simulink model "vhs_fpga_rx_to_sdram_time_share_agc_cfo_4Chan"  (Simulink 7.1)
settings: Solver=FixedStepDiscrete  SolverMode=SingleTasking  StartTime=0.0  StopTime=120000  RelTol=1e-3
values from neighbouring files (symbols this model uses):
  Nfft = 64    [OFDM_Parameter.mat]
  Nguard = 16    [OFDM_Parameter.mat]
  Nofdm = 130    [OFDM_Parameter.mat]
  Nskip = 8    [OFDM_Parameter.mat]
undefined symbols (not defined in the file or in its folder): Fs, Sincos_Bits, Sincos_Len, Theta_Bits
libraries: xbsIndex_r4 x407, vhsadac_common_ob_fpgalib_v1_2_0 x18, misc_tools_fpgalib_v1_0_0 x6, rffe_fpgalib_v1_1_0 x1, rtdex_fpgalib_v1_1_0 x1
(part 3 of 5)

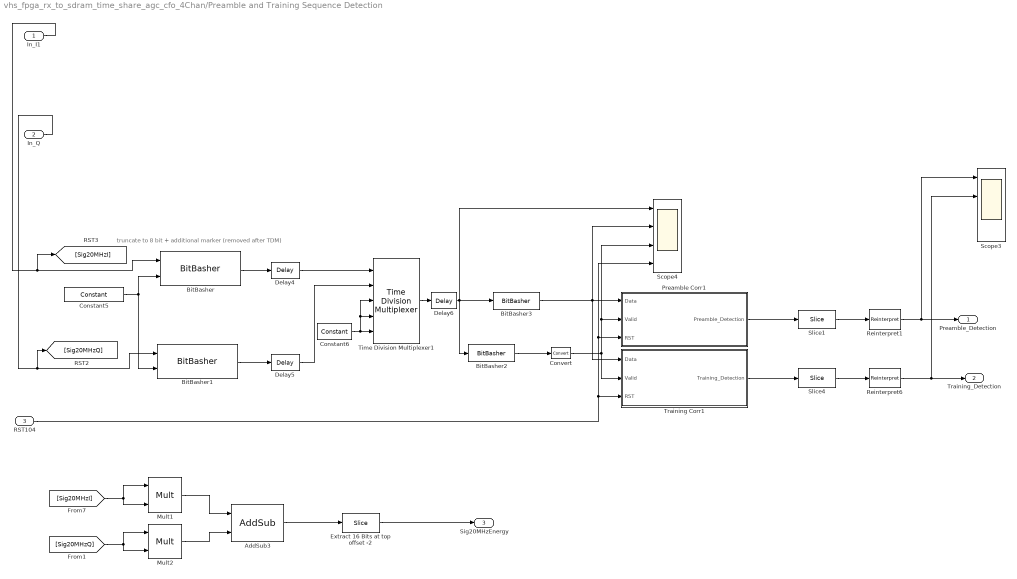
== system vhs_fpga_rx_to_sdram_time_share_agc_cfo_4Chan/Preamble and Training Sequence Detection ==
  note: truncate to 8 bit + additional marker (removed after TDM)
  In_I1 : Inport  OutDataType=sfix(16)  OutScaling=2^0
  In_Q : Inport  Port=2  OutDataType=sfix(16)  OutScaling=2^0
  RST104 : Inport  Port=3  OutDataType=sfix(16)  OutScaling=2^0
  "   Extract 16 Bits at top offset -2" : xbsIndex_r4/Slice  nbits=16  boolean_output=off  mode=Upper Bit Location + Width  bit1=-2  base1=MSB of Input  bit0=0  base0=LSB of Input  dbl_ovrd=off  block_type=slice
      settings: infoedit="Extracts a given range of bits from each input sample and presents it at the output.  The output type is ordinarily unsigned with binary point at zero, but can be Boolean when the slice is one bit wide.<P><P>Hardware notes: In hardware this block costs nothing."  block_version=10.1.3
  AddSub3 : xbsIndex_r4/AddSub  mode=Addition  use_carryin=off  use_carryout=off  en=off  latency=1  precision=Full  arith_type=Unsigned  n_bits=16  bin_pt=14  quantization=Truncate  overflow=Wrap  dbl_ovrd=off  use_behavioral_HDL=off  pipelined=off  use_rpm=on  hw_selection=Fabric  block_type=addsub
      settings: block_version=10.1.3
  BitBasher : xbsIndex_r4/BitBasher  bitexpr=|  display_expr=on  sr_1=1  arith_type1="Signed  (2's comp)"  bin_pt1=0  sr_2=2  arith_type2=Unsigned  bin_pt2=0  sr_3=3  arith_type3=Unsigned  bin_pt3=0  sr_4=4  arith_type4=Unsigned  bin_pt4=0  dbl_ovrd=off  block_type=bitbasher
      | <html><head><meta name="qrichtext" content="1" /><style type="text/css">
      | p, li { white-space: pre-wrap; }
      | </style></head><body style=" font-family:'MS Shell Dlg 2'; font-size:8.25pt; font-weight:400; font-style:normal;">
      | <p style=" margin-top:12px; margin-bottom:12px; margin-left:0px; margin-right:0px; -qt-block-indent:0; text-indent:0px; font-family:'MS Shell Dlg'; font-size:8pt;">a={b[13:6],c}</p></body></html>
      settings: block_version=10.1.3
  BitBasher1 : xbsIndex_r4/BitBasher  bitexpr=|  display_expr=on  sr_1=1  arith_type1="Signed  (2's comp)"  bin_pt1=0  sr_2=2  arith_type2=Unsigned  bin_pt2=0  sr_3=3  arith_type3=Unsigned  bin_pt3=0  sr_4=4  arith_type4=Unsigned  bin_pt4=0  dbl_ovrd=off  block_type=bitbasher
      | <html><head><meta name="qrichtext" content="1" /><style type="text/css">
      | p, li { white-space: pre-wrap; }
      | </style></head><body style=" font-family:'MS Shell Dlg 2'; font-size:8.25pt; font-weight:400; font-style:normal;">
      | <p style=" margin-top:12px; margin-bottom:12px; margin-left:0px; margin-right:0px; -qt-block-indent:0; text-indent:0px; font-family:'MS Shell Dlg'; font-size:8pt;">a={b[13:6],c}</p></body></html>
      settings: block_version=10.1.3
  BitBasher2 : xbsIndex_r4/BitBasher  bitexpr=|  display_expr=on  sr_1=1  arith_type1=Unsigned  bin_pt1=0  sr_2=2  arith_type2=Unsigned  bin_pt2=0  sr_3=3  arith_type3=Unsigned  bin_pt3=0  sr_4=4  arith_type4=Unsigned  bin_pt4=0  dbl_ovrd=off  block_type=bitbasher
      | <html><head><meta name="qrichtext" content="1" /><style type="text/css">
      | p, li { white-space: pre-wrap; }
      | </style></head><body style=" font-family:'MS Shell Dlg 2'; font-size:8.25pt; font-weight:400; font-style:normal;">
      | <p style=" margin-top:12px; margin-bottom:12px; margin-left:0px; margin-right:0px; -qt-block-indent:0; text-indent:0px; font-family:'MS Shell Dlg'; font-size:8pt;">a={b[0]}</p></body></html>
      settings: block_version=10.1.3
  BitBasher3 : xbsIndex_r4/BitBasher  bitexpr=|  display_expr=on  sr_1=1  arith_type1="Signed  (2's comp)"  bin_pt1=0  sr_2=2  arith_type2=Unsigned  bin_pt2=0  sr_3=3  arith_type3=Unsigned  bin_pt3=0  sr_4=4  arith_type4=Unsigned  bin_pt4=0  dbl_ovrd=off  block_type=bitbasher
      | <html><head><meta name="qrichtext" content="1" /><style type="text/css">
      | p, li { white-space: pre-wrap; }
      | </style></head><body style=" font-family:'MS Shell Dlg 2'; font-size:8.25pt; font-weight:400; font-style:normal;">
      | <p style=" margin-top:12px; margin-bottom:12px; margin-left:0px; margin-right:0px; -qt-block-indent:0; text-indent:0px; font-family:'MS Shell Dlg'; font-size:8pt;">a={b[8:1]}</p></body></html>
      settings: block_version=10.1.3
  Constant5 : xbsIndex_r4/Constant  arith_type=Unsigned  const=1  n_bits=1  bin_pt=0  explicit_period=on  period=5  equ=P=C  opselect=C  inp2=PCIN>>17  opr=+  inp1=P  carry=CIN  dbl_ovrd=off  block_type=constant
  Constant6 : xbsIndex_r4/Constant  arith_type=Signed (2's comp)  const=0  n_bits=9  bin_pt=0  explicit_period=on  period=5  equ=P=C  opselect=C  inp2=PCIN>>17  opr=+  inp1=P  carry=CIN  dbl_ovrd=off  block_type=constant
  Convert : xbsIndex_r4/Convert  arith_type=Boolean  n_bits=16  bin_pt=14  quantization=Truncate  overflow=Wrap  latency=0  dbl_ovrd=off  pipeline=off  block_type=convert
      settings: block_version=10.1.3
  Delay4 : xbsIndex_r4/Delay  en=off  latency=1  dbl_ovrd=off  reg_retiming=off  block_type=delay
  Delay5 : xbsIndex_r4/Delay  en=off  latency=1  dbl_ovrd=off  reg_retiming=off  block_type=delay
  Delay6 : xbsIndex_r4/Delay  en=off  latency=1  dbl_ovrd=off  reg_retiming=off  block_type=delay
  Mult1 : xbsIndex_r4/Mult  precision=Full  arith_type="Signed  (2's comp)"  n_bits=16  bin_pt=14  quantization=Truncate  overflow=Wrap  en=off  latency=3  dbl_ovrd=off  use_behavioral_HDL=off  use_embedded=on  opt=Speed  optimum_pipeline=off  pipeline=on  use_rpm=on  placement_style=Triangular  block_type=mult
      settings: infoedit=Hardware notes: To use the internal pipeline stage of the dedicated multiplier you must select 'Pipeline for maximum performance'.  block_version=10.1.3
  Mult2 : xbsIndex_r4/Mult  precision=Full  arith_type="Signed  (2's comp)"  n_bits=16  bin_pt=14  quantization=Truncate  overflow=Wrap  en=off  latency=3  dbl_ovrd=off  use_behavioral_HDL=off  use_embedded=on  opt=Speed  optimum_pipeline=off  pipeline=on  use_rpm=on  placement_style=Triangular  block_type=mult
      settings: infoedit=Hardware notes: To use the internal pipeline stage of the dedicated multiplier you must select 'Pipeline for maximum performance'.  block_version=10.1.3
  Preamble Corr1 : Subsystem
  Reinterpret1 : xbsIndex_r4/Reinterpret  force_arith_type=on  arith_type=Unsigned  force_bin_pt=on  bin_pt=0  block_type=reinterpret
      settings: infoedit="Changes signal type without altering the binary representation.   You can changed the signal between signed and unsigned, and relocate the binary point.<P><P>Hardware notes: In hardware this block costs nothing.<P><P>Example:  Suppose the input is 6 bits wide, signed, with 2 fractional bits, and the output is forced to unsigned with 0 fractional bits.  Then an input of -2.0 (1110.00 in binary 2's complement) becomes an output of 56 (111000 in binary)."  block_version=10.1.3
  Reinterpret6 : xbsIndex_r4/Reinterpret  force_arith_type=on  arith_type=Unsigned  force_bin_pt=on  bin_pt=0  block_type=reinterpret
      settings: infoedit="Changes signal type without altering the binary representation.   You can changed the signal between signed and unsigned, and relocate the binary point.<P><P>Hardware notes: In hardware this block costs nothing.<P><P>Example:  Suppose the input is 6 bits wide, signed, with 2 fractional bits, and the output is forced to unsigned with 0 fractional bits.  Then an input of -2.0 (1110.00 in binary 2's complement) becomes an output of 56 (111000 in binary)."  block_version=10.1.3
  Scope3 : Scope  NumInputPorts=4
      settings: YMin=-5~-5~-5~-5  YMax=5~5~5~5  SaveName=ScopeData5  MaxDataPoints=500000  SampleInput=on
  Scope4 : Scope  NumInputPorts=4
      settings: YMin=-300~-150~0~-1  YMax=200~100~1~1  SaveName=ScopeData10  MaxDataPoints=500000
  Slice1 : xbsIndex_r4/Slice  nbits=16  boolean_output=off  mode=Upper Bit Location + Width  bit1=-8  base1=MSB of Input  bit0=0  base0=LSB of Input  dbl_ovrd=off  block_type=slice
      settings: infoedit="Extracts a given range of bits from each input sample and presents it at the output.  The output type is ordinarily unsigned with binary point at zero, but can be Boolean when the slice is one bit wide.<P><P>Hardware notes: In hardware this block costs nothing."  block_version=10.1.3
  Slice4 : xbsIndex_r4/Slice  nbits=16  boolean_output=off  mode=Upper Bit Location + Width  bit1=-7  base1=MSB of Input  bit0=0  base0=LSB of Input  dbl_ovrd=off  block_type=slice
      settings: infoedit="Extracts a given range of bits from each input sample and presents it at the output.  The output type is ordinarily unsigned with binary point at zero, but can be Boolean when the slice is one bit wide.<P><P>Hardware notes: In hardware this block costs nothing."  block_version=10.1.3
  Time Division Multiplexer1 : xbsIndex_r4/Time Division Multiplexer  inputs=5  vin=off  dbl_ovrd=off  explicit_period=off  period=1  block_type=tdm
      settings: infoedit="Multiple inputs are sampled and  presented serially at the output."  block_version=10.1.3
  Training Corr1 : Subsystem
  Preamble_Detection : Outport  OutDataType=sfix(16)  OutScaling=2^0
  Training_Detection : Outport  Port=2  OutDataType=sfix(16)  OutScaling=2^0
  Sig20MHzEnergy : Outport  Port=3  OutDataType=sfix(16)  OutScaling=2^0
  wires:
  In_Q/1 -> BitBasher1/1, [Sig20MHzQ]
  In_I1/1 -> BitBasher/1, [Sig20MHzI]
  [Sig20MHzI] -> Mult1/1, Mult1/2
  [Sig20MHzQ] -> Mult2/2, Mult2/1
  Mult1/1 -> AddSub3/1
  Mult2/1 -> AddSub3/2
  AddSub3/1 -> "   Extract 16 Bits at top offset -2"/1
  "   Extract 16 Bits at top offset -2"/1 -> Sig20MHzEnergy/1
  Time Division Multiplexer1/1 -> Delay6/1
  Constant6/1 -> Time Division Multiplexer1/5, Time Division Multiplexer1/4, Time Division Multiplexer1/3
  BitBasher2/1 -> Convert/1
  Constant5/1 -> BitBasher/2, BitBasher1/2
  BitBasher1/1 -> Delay5/1
  BitBasher3/1 -> Preamble Corr1/1(Data), Training Corr1/1(Data), Scope4/2
  BitBasher/1 -> Delay4/1
  Convert/1 -> Training Corr1/2(Valid), Preamble Corr1/2(Valid), Scope4/3
  Preamble Corr1/1(Preamble_Detection) -> Slice1/1
  Slice1/1 -> Reinterpret1/1
  Delay4/1 -> Time Division Multiplexer1/1
  Delay5/1 -> Time Division Multiplexer1/2
  Delay6/1 -> BitBasher3/1, BitBasher2/1, Scope4/1
  Slice4/1 -> Reinterpret6/1
  Training Corr1/1(Training_Detection) -> Slice4/1
  Reinterpret6/1 -> Training_Detection/1, Scope3/2
  Reinterpret1/1 -> Preamble_Detection/1, Scope3/1
  RST104/1 -> Training Corr1/3(RST), Preamble Corr1/3(RST), Scope4/4

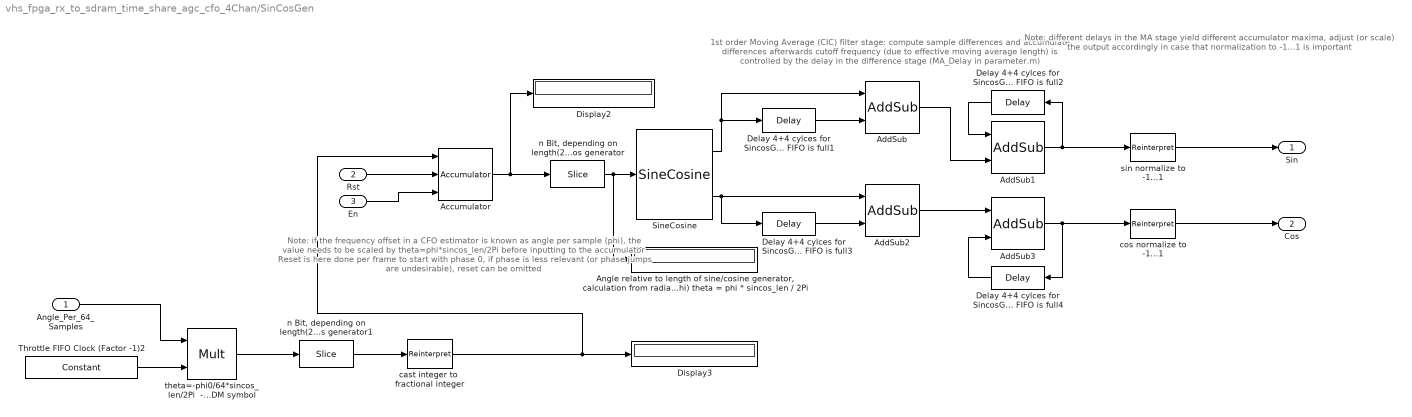
== system vhs_fpga_rx_to_sdram_time_share_agc_cfo_4Chan/SinCosGen ==
  note: 1st order Moving Average (CIC) filter stage:
      | compute sample differences and accumulate differences afterwards
      | cutoff frequency (due to effective moving average length) is
      | controlled by the delay in the difference stage (MA_Delay in parameter.m)
  note: Note: if the frequency offset in a CFO estimator
      | is known as angle per sample (phi),
      | the value needs to be scaled by
      | theta=phi*sincos_len/2Pi
      | before inputting to the accumulator
      | Reset is here done per frame to start with phase 0,
      | if phase is less relevant (or phase jumps are undesirable),
      | reset can be omitted
  note: Note: different delays in the MA stage yield different
      | accumulator maxima, adjust (or scale) the output accordingly
      | in case that normalization to -1...1 is important
  Angle_Per_64_Samples : Inport
  Rst : Inport  Port=2
  En : Inport  Port=3
  Accumulator : xbsIndex_r4/Accumulator  operation=Add  n_bits=Theta_Bits+Sincos_Bits+1  overflow=Wrap  scale=1  rst=on  hasbypass=off  en=on  dbl_ovrd=off  use_behavioral_HDL=on  implementation=Fabric  block_type=accum
      settings: infoedit="Adder or subtractor-based accumulator.   Output type and binary point position match the input.<P><P>Hardware notes: When \"Reinitialize with input 'b' on reset\" is selected, the accumulator is forced to run at the system rate even if the input 'b' is running at a slower rate."  block_version=10.1.3
  AddSub : xbsIndex_r4/AddSub  mode=Subtraction  use_carryin=off  use_carryout=off  en=off  latency=0  precision=Full  arith_type=Unsigned  n_bits=16  bin_pt=14  quantization=Truncate  overflow=Wrap  dbl_ovrd=off  use_behavioral_HDL=off  pipelined=off  use_rpm=on  hw_selection=Fabric  block_type=addsub
      settings: block_version=10.1.3
  AddSub1 : xbsIndex_r4/AddSub  mode=Addition  use_carryin=off  use_carryout=off  en=off  latency=0  precision=User Defined  arith_type="Signed  (2's comp)"  n_bits=16  bin_pt=8  quantization=Truncate  overflow=Wrap  dbl_ovrd=off  use_behavioral_HDL=off  pipelined=off  use_rpm=on  hw_selection=Fabric  block_type=addsub
      settings: block_version=10.1.3
  AddSub2 : xbsIndex_r4/AddSub  mode=Subtraction  use_carryin=off  use_carryout=off  en=off  latency=0  precision=Full  arith_type=Unsigned  n_bits=16  bin_pt=14  quantization=Truncate  overflow=Wrap  dbl_ovrd=off  use_behavioral_HDL=off  pipelined=off  use_rpm=on  hw_selection=Fabric  block_type=addsub
      settings: block_version=10.1.3
  AddSub3 : xbsIndex_r4/AddSub  mode=Addition  use_carryin=off  use_carryout=off  en=off  latency=0  precision=User Defined  arith_type="Signed  (2's comp)"  n_bits=16  bin_pt=8  quantization=Truncate  overflow=Wrap  dbl_ovrd=off  use_behavioral_HDL=off  pipelined=off  use_rpm=on  hw_selection=Fabric  block_type=addsub
      settings: block_version=10.1.3
  "Angle relative to length of sine/cosine generator, calculation from radians (phi) theta = phi * sincos_len / 2Pi" : Display
  Delay 4+4 cylces for SincosGen (Counter+Mult+SinCos latencies)  but stop immediately when FIFO is full1 : xbsIndex_r4/Delay  en=off  latency=MA_Delay  dbl_ovrd=off  reg_retiming=off  block_type=delay
  Delay 4+4 cylces for SincosGen (Counter+Mult+SinCos latencies)  but stop immediately when FIFO is full2 : xbsIndex_r4/Delay  Orientation=left  en=off  latency=1  dbl_ovrd=off  reg_retiming=off  block_type=delay
  Delay 4+4 cylces for SincosGen (Counter+Mult+SinCos latencies)  but stop immediately when FIFO is full3 : xbsIndex_r4/Delay  en=off  latency=MA_Delay  dbl_ovrd=off  reg_retiming=off  block_type=delay
  Delay 4+4 cylces for SincosGen (Counter+Mult+SinCos latencies)  but stop immediately when FIFO is full4 : xbsIndex_r4/Delay  Orientation=left  en=off  latency=1  dbl_ovrd=off  reg_retiming=off  block_type=delay
  Display2 : Display
  Display3 : Display
  SineCosine : xbsIndex_r4/SineCosine  mode=Sine and Cosine  neg_sin=off  neg_cos=off  n_bits=10  sym_output=on  en=off  latency=Sincos_Latency  dbl_ovrd=off  explicit_period=on  period=FreqDivider  mem_type=Distributed Memory  pipeline=off  use_rpm=on  block_type=sincos
      settings: block_version=10.1.3
  Throttle FIFO Clock (Factor -1)2 : xbsIndex_r4/Constant  arith_type=Signed (2's comp)  const=-1/64*Sincos_Len/(2*pi)  n_bits=32  bin_pt=28  explicit_period=on  period=5  equ=P=C  opselect=C  inp2=PCIN>>17  opr=+  inp1=P  carry=CIN  dbl_ovrd=off  block_type=constant
  cast integer to  fractional integer : xbsIndex_r4/Reinterpret  force_arith_type=on  arith_type="Signed  (2's comp)"  force_bin_pt=on  bin_pt=Theta_Bits  block_type=reinterpret
      settings: infoedit="Changes signal type without altering the binary representation.   You can changed the signal between signed and unsigned, and relocate the binary point.<P><P>Hardware notes: In hardware this block costs nothing.<P><P>Example:  Suppose the input is 6 bits wide, signed, with 2 fractional bits, and the output is forced to unsigned with 0 fractional bits.  Then an input of -2.0 (1110.00 in binary 2's complement) becomes an output of 56 (111000 in binary)."  block_version=10.1.3
  cos normalize to -1...1 : xbsIndex_r4/Reinterpret  force_arith_type=on  arith_type="Signed  (2's comp)"  force_bin_pt=on  bin_pt=14  block_type=reinterpret
      settings: infoedit="Changes signal type without altering the binary representation.   You can changed the signal between signed and unsigned, and relocate the binary point.<P><P>Hardware notes: In hardware this block costs nothing.<P><P>Example:  Suppose the input is 6 bits wide, signed, with 2 fractional bits, and the output is forced to unsigned with 0 fractional bits.  Then an input of -2.0 (1110.00 in binary 2's complement) becomes an output of 56 (111000 in binary)."  block_version=10.1.3
  "n Bit, depending on length(2^n) of sincos generator" : xbsIndex_r4/Slice  nbits=Sincos_Bits  boolean_output=off  mode=Lower Bit Location + Width  bit1=0  base1=MSB of Input  bit0=Theta_Bits  base0=LSB of Input  dbl_ovrd=off  block_type=slice
      settings: infoedit="Extracts a given range of bits from each input sample and presents it at the output.  The output type is ordinarily unsigned with binary point at zero, but can be Boolean when the slice is one bit wide.<P><P>Hardware notes: In hardware this block costs nothing."  block_version=10.1.3
  "n Bit, depending on length(2^n) of sincos generator1" : xbsIndex_r4/Slice  nbits=32  boolean_output=off  mode=Upper Bit Location + Width  bit1=0  base1=MSB of Input  bit0=Theta_Bits  base0=LSB of Input  dbl_ovrd=off  block_type=slice
      settings: infoedit="Extracts a given range of bits from each input sample and presents it at the output.  The output type is ordinarily unsigned with binary point at zero, but can be Boolean when the slice is one bit wide.<P><P>Hardware notes: In hardware this block costs nothing."  block_version=10.1.3
  sin normalize to -1...1 : xbsIndex_r4/Reinterpret  force_arith_type=on  arith_type="Signed  (2's comp)"  force_bin_pt=on  bin_pt=14  block_type=reinterpret
      settings: infoedit="Changes signal type without altering the binary representation.   You can changed the signal between signed and unsigned, and relocate the binary point.<P><P>Hardware notes: In hardware this block costs nothing.<P><P>Example:  Suppose the input is 6 bits wide, signed, with 2 fractional bits, and the output is forced to unsigned with 0 fractional bits.  Then an input of -2.0 (1110.00 in binary 2's complement) becomes an output of 56 (111000 in binary)."  block_version=10.1.3
  "theta=-phi0/64*sincos_len/2Pi  -> /64: CFO is for a distance of 64 samples between guard interval and main OFDM symbol" : xbsIndex_r4/Mult  precision=Full  arith_type="Signed  (2's comp)"  n_bits=16  bin_pt=14  quantization=Truncate  overflow=Wrap  en=off  latency=3  dbl_ovrd=off  use_behavioral_HDL=off  use_embedded=on  opt=Speed  optimum_pipeline=off  pipeline=on  use_rpm=on  placement_style=Triangular  block_type=mult
      settings: infoedit=Hardware notes: To use the internal pipeline stage of the dedicated multiplier you must select 'Pipeline for maximum performance'.  block_version=10.1.3
  Sin : Outport
  Cos : Outport  Port=2
  wires:
  "n Bit, depending on length(2^n) of sincos generator"/1 -> SineCosine/1, "Angle relative to length of sine/cosine generator, calculation from radians (phi) theta = phi * sincos_len / 2Pi"/1
  SineCosine/1 -> Delay 4+4 cylces for SincosGen (Counter+Mult+SinCos latencies)  but stop immediately when FIFO is full1/1, AddSub/1
  SineCosine/2 -> AddSub2/1, Delay 4+4 cylces for SincosGen (Counter+Mult+SinCos latencies)  but stop immediately when FIFO is full3/1
  Accumulator/1 -> "n Bit, depending on length(2^n) of sincos generator"/1, Display2/1
  cast integer to  fractional integer/1 -> Display3/1, Accumulator/1
  AddSub1/1 -> Delay 4+4 cylces for SincosGen (Counter+Mult+SinCos latencies)  but stop immediately when FIFO is full2/1, sin normalize to -1...1/1
  Delay 4+4 cylces for SincosGen (Counter+Mult+SinCos latencies)  but stop immediately when FIFO is full2/1 -> AddSub1/1
  Delay 4+4 cylces for SincosGen (Counter+Mult+SinCos latencies)  but stop immediately when FIFO is full3/1 -> AddSub2/2
  AddSub2/1 -> AddSub3/1
  AddSub3/1 -> Delay 4+4 cylces for SincosGen (Counter+Mult+SinCos latencies)  but stop immediately when FIFO is full4/1, cos normalize to -1...1/1
  Delay 4+4 cylces for SincosGen (Counter+Mult+SinCos latencies)  but stop immediately when FIFO is full4/1 -> AddSub3/2
  AddSub/1 -> AddSub1/2
  Delay 4+4 cylces for SincosGen (Counter+Mult+SinCos latencies)  but stop immediately when FIFO is full1/1 -> AddSub/2
  Rst/1 -> Accumulator/2
  Throttle FIFO Clock (Factor -1)2/1 -> "theta=-phi0/64*sincos_len/2Pi  -> /64: CFO is for a distance of 64 samples between guard interval and main OFDM symbol"/2
  "theta=-phi0/64*sincos_len/2Pi  -> /64: CFO is for a distance of 64 samples between guard interval and main OFDM symbol"/1 -> "n Bit, depending on length(2^n) of sincos generator1"/1
  "n Bit, depending on length(2^n) of sincos generator1"/1 -> cast integer to  fractional integer/1
  Angle_Per_64_Samples/1 -> "theta=-phi0/64*sincos_len/2Pi  -> /64: CFO is for a distance of 64 samples between guard interval and main OFDM symbol"/1
  sin normalize to -1...1/1 -> Sin/1
  cos normalize to -1...1/1 -> Cos/1
  En/1 -> Accumulator/3

== system vhs_fpga_rx_to_sdram_time_share_agc_cfo_4Chan/two times  long preamble detection ==
  note: original delay: (Nfft+Nguard)
      | due to shortened Training Correlator: Nfft-16
  Preamble Detection : Inport  OutDataType=sfix(16)  OutScaling=2^0
  Training Detection : Inport  Port=2  OutDataType=sfix(16)  OutScaling=2^0
  Delay1 : xbsIndex_r4/Delay  en=off  latency=48  dbl_ovrd=off  reg_retiming=off  block_type=delay
      settings: block_version=9.2.00
  Edge detector : misc_tools_fpgalib_v1_0_0/Edge detector  Tag=LYR_FPGA_MISC_EDGE_DETECTOR  Description=Lyrtech block  SystemSampleTime=-1  edge_detect=Rising  and_latency=0
  Expression6 : xbsIndex_r4/Expression  expression=a & b  align_bp=on  en=off  latency=0  precision=Full  arith_type=Unsigned  n_bits=16  bin_pt=0  dbl_ovrd=off  block_type=expr
      settings: block_version=10.1.3
  Detected : Outport  OutDataType=sfix(16)  OutScaling=2^0
  wires:
  Preamble Detection/1 -> Delay1/1
  Expression6/1 -> Edge detector/1
  Edge detector/1 -> Detected/1
  Training Detection/1 -> Expression6/2
  Delay1/1 -> Expression6/1

== system vhs_fpga_rx_to_sdram_time_share_agc_cfo_4Chan/CFO Estimate - triggered by WRITE_STATE going high/CORDIC ATAN1 ==
  note: The CORDIC algorithm is implemented in 3 steps.
      |
      | Step 1: Coarse Angle Rotation.  The algorithm converges only for angles between -pi/2 and pi/2, so if x < zero, the input vector is reflected
      | to the 1st or 3rd quadrant by making the x-coordinate non-negative.
      |
      | Step 2: Fine Angle Rotation.  For rectangular-to-polar conversion, the resulting vector is rotated through progressively smaller angles, such that y goes
      | to zero. In the i-th stage, the angular rotation is by either +/- atan(1/2^i), depending on whether or not its input y is less than or greater than zero.
      |
      | Step 3: Angle Correction. If there was a reflection applied in Step 1, this step applies the appropriate angle correction by subtracting it from +/- pi.
  x : Inport  OutDataType=sfix(16)  OutScaling=2^0
  y : Inport  Port=2  OutDataType=sfix(16)  OutScaling=2^0
  CORDIC  Pipe Balance : xbsIndex_r4/Delay  en=off  latency=sum(pipeline)  dbl_ovrd=off  reg_retiming=off  block_type=delay
      settings: infoedit="Delay line having  configurable length.<P><P>Hardware notes: A delay line is a chain, each link of which is an SRL16 followed by a flip-flop. If register retiming is enabled, the delay line is a chain of flip-flops."  xl_area=[0, 0, 0, 0, 0, 0, 0]  block_version=VER_STRING_GOES_HERE
  CORDIC  Pipe Balance1 : xbsIndex_r4/Delay  en=off  latency=sum(pipeline)+1  dbl_ovrd=off  reg_retiming=off  block_type=delay
      settings: infoedit="Delay line having  configurable length.<P><P>Hardware notes: A delay line is a chain, each link of which is an SRL16 followed by a flip-flop. If register retiming is enabled, the delay line is a chain of flip-flops."  xl_area=[0, 0, 0, 0, 0, 0, 0]  block_version=VER_STRING_GOES_HERE
  CORDIC  Pipe Balance2 : xbsIndex_r4/Delay  en=off  latency=1  dbl_ovrd=off  reg_retiming=off  block_type=delay
      settings: infoedit="Delay line having  configurable length.<P><P>Hardware notes: A delay line is a chain, each link of which is an SRL16 followed by a flip-flop. If register retiming is enabled, the delay line is a chain of flip-flops."  xl_area=[0, 0, 0, 0, 0, 0, 0]  block_version=VER_STRING_GOES_HERE
  CORDIC Fine Angle PE : Subsystem  mask(CORDIC parallel PE){}
      mask init:
      | [bg,fg] = xlcmap('XBlock',0);
      | iPos = get_param(gcb,'Position');
      | iWidth=iPos(3)-iPos(1); iHeight=iPos(4)-iPos(2);
      | iCx=iWidth/2;
      | iCy=iHeight/2;
      | [logoX, logoY] = xlogo(iPos);
      mask Display:
      | patch([0 iWidth iWidth 0],[0 0 iHeight iHeight] , bg);
      | patch(logoX,logoY , fg);
      | port_label('input',1,'x');
      | port_label('input',2,'y');
      | port_label('input',3,'z');
      | port_label('output',1,'X');
      | port_label('output',2,'Z');
      | plot([0 0 iWidth iWidth 0], [0 iHeight iHeight 0 0]);
  Constant : xbsIndex_r4/Constant  arith_type=Signed (2's comp)  const=0  n_bits=pe_nbits  bin_pt=pe_binpt  explicit_period=off  period=1  equ=P=C  opselect=C  inp2=PCIN>>17  opr=+  inp1=P  carry=CIN  dbl_ovrd=off  block_type=constant
      settings: block_version=VER_STRING_GOES_HERE
  Quadrant Correct : Subsystem
      mask init:
      | [bg,fg] = xlcmap('XBlock',0);
      | iPos = get_param(gcb,'Position');
      | iWidth=iPos(3)-iPos(1); iHeight=iPos(4)-iPos(2);
      | iCx=iWidth/2;
      | iCy=iHeight/2;
      | [logoX, logoY] = xlogo(iPos);
      mask Display:
      | patch([0 iWidth iWidth 0],[0 0 iHeight iHeight] , bg);
      | patch(logoX,logoY , fg);
      | port_label('input',1,'Z in');
      | port_label('input',2,'sgn(y)');
      | port_label('input',3,'sgn(x)');
      | port_label('output',1,'Z');
      | plot([0 0 iWidth iWidth 0], [0 iHeight iHeight 0 0]);
  Quadrant Map : Subsystem
      mask init:
      | [bg,fg] = xlcmap('XBlock',0);
      | iPos = get_param(gcb,'Position');
      | iWidth=iPos(3)-iPos(1); iHeight=iPos(4)-iPos(2);
      | iCx=iWidth/2;
      | iCy=iHeight/2;
      | [logoX, logoY] = xlogo(iPos);
      mask Display:
      | patch([0 iWidth iWidth 0],[0 0 iHeight iHeight] , bg);
      | patch(logoX,logoY , fg);
      | port_label('input',1,'x');
      | port_label('input',2,'y');
      | port_label('output',1,'X');
      | port_label('output',2,'Y');
      | port_label('output',3,'sgn(y)');
      | port_label('output',4,'sgn(x)');
      | plot([0 0 iWidth iWidth 0], [0 iHeight iHeight 0 0]);
  X : Outport  OutDataType=sfix(16)  OutScaling=2^0
  Z : Outport  Port=2  OutDataType=sfix(16)  OutScaling=2^0
  wires:
  CORDIC  Pipe Balance2/1 -> X/1
  CORDIC Fine Angle PE/1(X) -> CORDIC  Pipe Balance2/1
  Quadrant Correct/1(Z) -> Z/1
  CORDIC Fine Angle PE/2(Z) -> Quadrant Correct/1(Z IN)
  CORDIC  Pipe Balance1/1 -> Quadrant Correct/3(Z MUX SEL)
  CORDIC  Pipe Balance/1 -> Quadrant Correct/2(PI_ addsub)
  Quadrant Map/4(sign(x)) -> CORDIC  Pipe Balance1/1
  Quadrant Map/3(sign(y)) -> CORDIC  Pipe Balance/1
  y/1 -> Quadrant Map/2(y)
  x/1 -> Quadrant Map/1(x)
  Quadrant Map/2(Y) -> CORDIC Fine Angle PE/2(y)
  Quadrant Map/1(X) -> CORDIC Fine Angle PE/1(x)
  Constant/1 -> CORDIC Fine Angle PE/3(z)

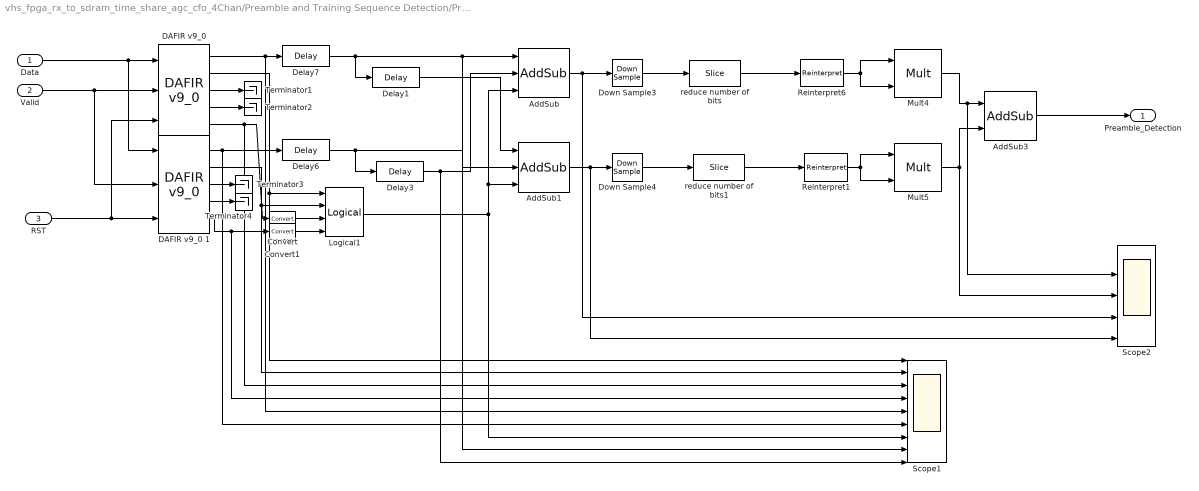
== system vhs_fpga_rx_to_sdram_time_share_agc_cfo_4Chan/Preamble and Training Sequence Detection/Preamble Corr1 ==
  Data : Inport  OutDataType=sfix(16)  OutScaling=2^0
  Valid : Inport  Port=2  OutDataType=sfix(16)  OutScaling=2^0
  RST : Inport  Port=3  OutDataType=sfix(16)  OutScaling=2^0
  AddSub : xbsIndex_r4/AddSub  mode=Addition  use_carryin=off  use_carryout=off  en=on  latency=1  precision=Full  arith_type=Unsigned  n_bits=16  bin_pt=14  quantization=Truncate  overflow=Wrap  dbl_ovrd=off  use_behavioral_HDL=off  pipelined=off  use_rpm=on  hw_selection=Fabric  block_type=addsub
      settings: block_version=10.1.3
  AddSub1 : xbsIndex_r4/AddSub  mode=Subtraction  use_carryin=off  use_carryout=off  en=on  latency=1  precision=Full  arith_type=Unsigned  n_bits=16  bin_pt=14  quantization=Truncate  overflow=Wrap  dbl_ovrd=off  use_behavioral_HDL=off  pipelined=off  use_rpm=on  hw_selection=Fabric  block_type=addsub
      settings: block_version=10.1.3
  AddSub3 : xbsIndex_r4/AddSub  mode=Addition  use_carryin=off  use_carryout=off  en=off  latency=1  precision=Full  arith_type=Unsigned  n_bits=16  bin_pt=14  quantization=Truncate  overflow=Wrap  dbl_ovrd=off  use_behavioral_HDL=off  pipelined=off  use_rpm=on  hw_selection=Fabric  block_type=addsub
      settings: block_version=10.1.3
  Convert : xbsIndex_r4/Convert  arith_type=Boolean  n_bits=16  bin_pt=14  quantization=Truncate  overflow=Wrap  latency=0  dbl_ovrd=off  pipeline=off  block_type=convert
      settings: block_version=10.1.3
  Convert1 : xbsIndex_r4/Convert  arith_type=Boolean  n_bits=16  bin_pt=14  quantization=Truncate  overflow=Wrap  latency=0  dbl_ovrd=off  pipeline=off  block_type=convert
      settings: block_version=10.1.3
  "DAFIR v9_0 " : xbsIndex_r4/DAFIR v9_0   coef=2^7 * real( conj([(longPreamble_time(end:-1:end-Nguard+1)) (longPreamble_time(end:-1:1))]) )  structure=Inferred from Coefficients  coef_n_bits=9  coef_bin_pt=0  over_sample=1  reload=off  valids=on  rst=on  latency=11  num_channels=2  serial_input=on  polyphase_behavior="Single Rate:  sample in - sample out"  dbl_ovrd=off  explicit_period=off  period=1  use_isim=0  block_type=fir
      settings: infoedit="Hardware notes: Implemented using distributed arithmetic (DA).  The hardware over sampling rate determines the degree of parallelism.  A rate of one produces a fully parallel DA filter.  A rate of n (resp., n+1) for an n-bit input signal produces a fully serial implementation for a non-symmetric (resp., symmetric) impulse response.  Intermediate values produce implementations with intermediate levels of parallelism."  block_version=10.1.3
  DAFIR v9_0 1 : xbsIndex_r4/DAFIR v9_0   coef=2^7 * imag( conj([(longPreamble_time(end:-1:end-Nguard+1)) (longPreamble_time(end:-1:1))]) )  structure=Inferred from Coefficients  coef_n_bits=9  coef_bin_pt=0  over_sample=1  reload=off  valids=on  rst=on  latency=11  num_channels=2  serial_input=on  polyphase_behavior="Single Rate:  sample in - sample out"  dbl_ovrd=off  explicit_period=off  period=1  use_isim=0  block_type=fir
      settings: infoedit="Hardware notes: Implemented using distributed arithmetic (DA).  The hardware over sampling rate determines the degree of parallelism.  A rate of one produces a fully parallel DA filter.  A rate of n (resp., n+1) for an n-bit input signal produces a fully serial implementation for a non-symmetric (resp., symmetric) impulse response.  Intermediate values produce implementations with intermediate levels of parallelism."  block_version=10.1.3
  Delay{1,3,6..7} (4 alike) : xbsIndex_r4/Delay  en=off  latency=1  dbl_ovrd=off  reg_retiming=off  block_type=delay
  Down Sample3 : xbsIndex_r4/Down Sample  sample_ratio=5  sample_phase="Last Value of Frame  (most efficient)"  en=off  latency=1  dbl_ovrd=off  block_type=dsamp
      settings: block_version=10.1.3
  Down Sample4 : xbsIndex_r4/Down Sample  sample_ratio=5  sample_phase="Last Value of Frame  (most efficient)"  en=off  latency=1  dbl_ovrd=off  block_type=dsamp
      settings: block_version=10.1.3
  Logical1 : xbsIndex_r4/Logical  logical_function=AND  inputs=4  en=off  latency=1  precision=Full  arith_type=Unsigned  n_bits=16  bin_pt=0  align_bp=on  dbl_ovrd=off  block_type=logical
  Mult4 : xbsIndex_r4/Mult  precision=Full  arith_type="Signed  (2's comp)"  n_bits=16  bin_pt=14  quantization=Truncate  overflow=Wrap  en=off  latency=3  dbl_ovrd=off  use_behavioral_HDL=off  use_embedded=on  opt=Speed  optimum_pipeline=off  pipeline=on  use_rpm=on  placement_style=Triangular  block_type=mult
      settings: infoedit=Hardware notes: To use the internal pipeline stage of the dedicated multiplier you must select 'Pipeline for maximum performance'.  block_version=10.1.3
  Mult5 : xbsIndex_r4/Mult  precision=Full  arith_type="Signed  (2's comp)"  n_bits=16  bin_pt=14  quantization=Truncate  overflow=Wrap  en=off  latency=3  dbl_ovrd=off  use_behavioral_HDL=off  use_embedded=on  opt=Speed  optimum_pipeline=off  pipeline=on  use_rpm=on  placement_style=Triangular  block_type=mult
      settings: infoedit=Hardware notes: To use the internal pipeline stage of the dedicated multiplier you must select 'Pipeline for maximum performance'.  block_version=10.1.3
  Reinterpret1 : xbsIndex_r4/Reinterpret  force_arith_type=on  arith_type="Signed  (2's comp)"  force_bin_pt=off  bin_pt=0  block_type=reinterpret
      settings: infoedit="Changes signal type without altering the binary representation.   You can changed the signal between signed and unsigned, and relocate the binary point.<P><P>Hardware notes: In hardware this block costs nothing.<P><P>Example:  Suppose the input is 6 bits wide, signed, with 2 fractional bits, and the output is forced to unsigned with 0 fractional bits.  Then an input of -2.0 (1110.00 in binary 2's complement) becomes an output of 56 (111000 in binary)."  block_version=10.1.3
  Reinterpret6 : xbsIndex_r4/Reinterpret  force_arith_type=on  arith_type="Signed  (2's comp)"  force_bin_pt=off  bin_pt=0  block_type=reinterpret
      settings: infoedit="Changes signal type without altering the binary representation.   You can changed the signal between signed and unsigned, and relocate the binary point.<P><P>Hardware notes: In hardware this block costs nothing.<P><P>Example:  Suppose the input is 6 bits wide, signed, with 2 fractional bits, and the output is forced to unsigned with 0 fractional bits.  Then an input of -2.0 (1110.00 in binary 2's complement) becomes an output of 56 (111000 in binary)."  block_version=10.1.3
  Scope1 : Scope  NumInputPorts=9
      settings: YMin=-200000~-500000~-200000~-500000~0~0~0~-5~-5  YMax=500000~200000~500000~200000~1~1~1~5~5  SaveName=ScopeData11  MaxDataPoints=500000
  Scope2 : Scope  NumInputPorts=5
      settings: YMin=-5~-5~-5~-5~-5  YMax=5~5~5~5~5  MaxDataPoints=500000
  Terminator{1..4} (4 alike) : Terminator
  reduce number of bits : xbsIndex_r4/Slice  nbits=20  boolean_output=off  mode=Upper Bit Location + Width  bit1=0  base1=MSB of Input  bit0=0  base0=LSB of Input  dbl_ovrd=off  block_type=slice
      settings: infoedit="Extracts a given range of bits from each input sample and presents it at the output.  The output type is ordinarily unsigned with binary point at zero, but can be Boolean when the slice is one bit wide.<P><P>Hardware notes: In hardware this block costs nothing."  block_version=10.1.3
  reduce number of bits1 : xbsIndex_r4/Slice  nbits=20  boolean_output=off  mode=Upper Bit Location + Width  bit1=0  base1=MSB of Input  bit0=0  base0=LSB of Input  dbl_ovrd=off  block_type=slice
      settings: infoedit="Extracts a given range of bits from each input sample and presents it at the output.  The output type is ordinarily unsigned with binary point at zero, but can be Boolean when the slice is one bit wide.<P><P>Hardware notes: In hardware this block costs nothing."  block_version=10.1.3
  Preamble_Detection : Outport  OutDataType=sfix(16)  OutScaling=2^0
  wires:
  DAFIR v9_0 1/4 -> Terminator4/1
  DAFIR v9_0 1/3 -> Terminator3/1
  "DAFIR v9_0 "/4 -> Terminator2/1
  "DAFIR v9_0 "/3 -> Terminator1/1
  Mult5/1 -> Scope2/3, AddSub3/2
  Mult4/1 -> Scope2/2, AddSub3/1
  Down Sample4/1 -> reduce number of bits1/1
  Down Sample3/1 -> reduce number of bits/1
  AddSub1/1 -> Scope2/5, Down Sample4/1
  AddSub/1 -> Down Sample3/1, Scope2/4
  AddSub3/1 -> Preamble_Detection/1
  Delay1/1 -> AddSub1/1
  RST/1 -> DAFIR v9_0 1/3, "DAFIR v9_0 "/3
  Data/1 -> DAFIR v9_0 1/1, "DAFIR v9_0 "/1
  Valid/1 -> "DAFIR v9_0 "/2, DAFIR v9_0 1/2
  Convert1/1 -> Logical1/4
  Convert/1 -> Logical1/3
  DAFIR v9_0 1/5 -> Convert1/1, Scope1/4
  "DAFIR v9_0 "/5 -> Convert/1, Scope1/3
  Logical1/1 -> AddSub/3, AddSub1/3, Scope1/7
  Delay3/1 -> AddSub/2, Scope1/9
  Delay6/1 -> AddSub1/2, Delay3/1
  Delay7/1 -> Delay1/1, AddSub/1, Scope1/8
  DAFIR v9_0 1/1 -> Delay6/1, Scope1/6
  "DAFIR v9_0 "/1 -> Delay7/1, Scope1/5
  DAFIR v9_0 1/2 -> Logical1/2, Scope1/2
  "DAFIR v9_0 "/2 -> Logical1/1, Scope1/1
  reduce number of bits/1 -> Reinterpret6/1
  reduce number of bits1/1 -> Reinterpret1/1
  Reinterpret6/1 -> Mult4/2, Mult4/1
  Reinterpret1/1 -> Mult5/2, Mult5/1

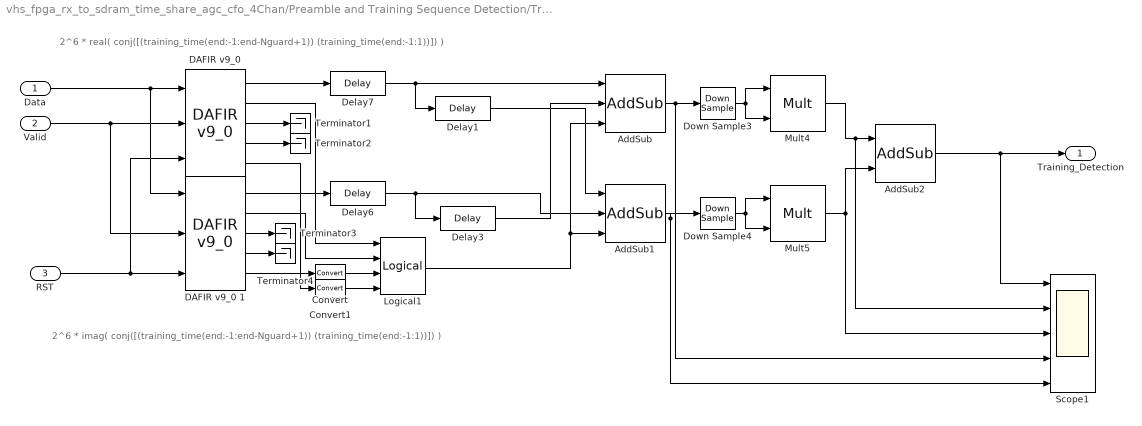
== system vhs_fpga_rx_to_sdram_time_share_agc_cfo_4Chan/Preamble and Training Sequence Detection/Training Corr1 ==
  note: 2^6 * real( conj([(training_time(end:-1:end-Nguard+1)) (training_time(end:-1:1))]) )
  note: 2^6 * imag( conj([(training_time(end:-1:end-Nguard+1)) (training_time(end:-1:1))]) )
  Data : Inport  OutDataType=sfix(16)  OutScaling=2^0
  Valid : Inport  Port=2  OutDataType=sfix(16)  OutScaling=2^0
  RST : Inport  Port=3  OutDataType=sfix(16)  OutScaling=2^0
  AddSub : xbsIndex_r4/AddSub  mode=Addition  use_carryin=off  use_carryout=off  en=on  latency=1  precision=Full  arith_type=Unsigned  n_bits=16  bin_pt=14  quantization=Truncate  overflow=Wrap  dbl_ovrd=off  use_behavioral_HDL=off  pipelined=off  use_rpm=on  hw_selection=Fabric  block_type=addsub
      settings: block_version=10.1.3
  AddSub1 : xbsIndex_r4/AddSub  mode=Subtraction  use_carryin=off  use_carryout=off  en=on  latency=1  precision=Full  arith_type=Unsigned  n_bits=16  bin_pt=14  quantization=Truncate  overflow=Wrap  dbl_ovrd=off  use_behavioral_HDL=off  pipelined=off  use_rpm=on  hw_selection=Fabric  block_type=addsub
      settings: block_version=10.1.3
  AddSub2 : xbsIndex_r4/AddSub  mode=Addition  use_carryin=off  use_carryout=off  en=off  latency=1  precision=Full  arith_type=Unsigned  n_bits=16  bin_pt=14  quantization=Truncate  overflow=Wrap  dbl_ovrd=off  use_behavioral_HDL=off  pipelined=off  use_rpm=on  hw_selection=Fabric  block_type=addsub
      settings: block_version=10.1.3
  Convert : xbsIndex_r4/Convert  arith_type=Boolean  n_bits=16  bin_pt=14  quantization=Truncate  overflow=Wrap  latency=0  dbl_ovrd=off  pipeline=off  block_type=convert
      settings: block_version=10.1.3
  Convert1 : xbsIndex_r4/Convert  arith_type=Boolean  n_bits=16  bin_pt=14  quantization=Truncate  overflow=Wrap  latency=0  dbl_ovrd=off  pipeline=off  block_type=convert
      settings: block_version=10.1.3
  "DAFIR v9_0 " : xbsIndex_r4/DAFIR v9_0   coef=2^6 * real( conj([(training_time(end-16:-1:1))]) )  structure=Inferred from Coefficients  coef_n_bits=9  coef_bin_pt=0  over_sample=1  reload=off  valids=on  rst=on  latency=11  num_channels=2  serial_input=on  polyphase_behavior="Single Rate:  sample in - sample out"  dbl_ovrd=off  explicit_period=off  period=1  use_isim=0  block_type=fir
      settings: infoedit="Hardware notes: Implemented using distributed arithmetic (DA).  The hardware over sampling rate determines the degree of parallelism.  A rate of one produces a fully parallel DA filter.  A rate of n (resp., n+1) for an n-bit input signal produces a fully serial implementation for a non-symmetric (resp., symmetric) impulse response.  Intermediate values produce implementations with intermediate levels of parallelism."  block_version=10.1.3
  DAFIR v9_0 1 : xbsIndex_r4/DAFIR v9_0   coef=2^6 * imag( conj([(training_time(end-16:-1:1))]) )  structure=Inferred from Coefficients  coef_n_bits=9  coef_bin_pt=0  over_sample=1  reload=off  valids=on  rst=on  latency=11  num_channels=2  serial_input=on  polyphase_behavior="Single Rate:  sample in - sample out"  dbl_ovrd=off  explicit_period=off  period=1  use_isim=0  block_type=fir
      settings: infoedit="Hardware notes: Implemented using distributed arithmetic (DA).  The hardware over sampling rate determines the degree of parallelism.  A rate of one produces a fully parallel DA filter.  A rate of n (resp., n+1) for an n-bit input signal produces a fully serial implementation for a non-symmetric (resp., symmetric) impulse response.  Intermediate values produce implementations with intermediate levels of parallelism."  block_version=10.1.3
  Delay{1,3,6..7} (4 alike) : xbsIndex_r4/Delay  en=off  latency=1  dbl_ovrd=off  reg_retiming=off  block_type=delay
  Down Sample3 : xbsIndex_r4/Down Sample  sample_ratio=5  sample_phase="Last Value of Frame  (most efficient)"  en=off  latency=1  dbl_ovrd=off  block_type=dsamp
      settings: block_version=10.1.3
  Down Sample4 : xbsIndex_r4/Down Sample  sample_ratio=5  sample_phase="Last Value of Frame  (most efficient)"  en=off  latency=1  dbl_ovrd=off  block_type=dsamp
      settings: block_version=10.1.3
  Logical1 : xbsIndex_r4/Logical  logical_function=AND  inputs=4  en=off  latency=1  precision=Full  arith_type=Unsigned  n_bits=16  bin_pt=0  align_bp=on  dbl_ovrd=off  block_type=logical
  Mult4 : xbsIndex_r4/Mult  precision=Full  arith_type="Signed  (2's comp)"  n_bits=16  bin_pt=14  quantization=Truncate  overflow=Wrap  en=off  latency=3  dbl_ovrd=off  use_behavioral_HDL=off  use_embedded=on  opt=Speed  optimum_pipeline=off  pipeline=on  use_rpm=on  placement_style=Triangular  block_type=mult
      settings: infoedit=Hardware notes: To use the internal pipeline stage of the dedicated multiplier you must select 'Pipeline for maximum performance'.  block_version=10.1.3
  Mult5 : xbsIndex_r4/Mult  precision=Full  arith_type="Signed  (2's comp)"  n_bits=16  bin_pt=14  quantization=Truncate  overflow=Wrap  en=off  latency=3  dbl_ovrd=off  use_behavioral_HDL=off  use_embedded=on  opt=Speed  optimum_pipeline=off  pipeline=on  use_rpm=on  placement_style=Triangular  block_type=mult
      settings: infoedit=Hardware notes: To use the internal pipeline stage of the dedicated multiplier you must select 'Pipeline for maximum performance'.  block_version=10.1.3
  Scope1 : Scope  NumInputPorts=5
      settings: YMin=-5~-5~-5~-5~-5  YMax=5~5~5~5~5  SaveName=ScopeData7  MaxDataPoints=500000
  Terminator{1..4} (4 alike) : Terminator
  Training_Detection : Outport  OutDataType=sfix(16)  OutScaling=2^0
  wires:
  DAFIR v9_0 1/4 -> Terminator4/1
  DAFIR v9_0 1/3 -> Terminator3/1
  "DAFIR v9_0 "/4 -> Terminator2/1
  "DAFIR v9_0 "/3 -> Terminator1/1
  Mult5/1 -> Scope1/3, AddSub2/2
  Mult4/1 -> Scope1/2, AddSub2/1
  Down Sample4/1 -> Mult5/2, Mult5/1
  Down Sample3/1 -> Mult4/2, Mult4/1
  AddSub1/1 -> Down Sample4/1, Scope1/5
  AddSub/1 -> Down Sample3/1, Scope1/4
  AddSub2/1 -> Training_Detection/1, Scope1/1
  Delay1/1 -> AddSub1/1
  RST/1 -> DAFIR v9_0 1/3, "DAFIR v9_0 "/3
  Data/1 -> DAFIR v9_0 1/1, "DAFIR v9_0 "/1
  Valid/1 -> "DAFIR v9_0 "/2, DAFIR v9_0 1/2
  Convert1/1 -> Logical1/4
  Convert/1 -> Logical1/3
  DAFIR v9_0 1/5 -> Convert1/1
  "DAFIR v9_0 "/5 -> Convert/1
  Logical1/1 -> AddSub/3, AddSub1/3
  Delay3/1 -> AddSub/2
  Delay6/1 -> AddSub1/2, Delay3/1
  Delay7/1 -> AddSub/1, Delay1/1
  DAFIR v9_0 1/1 -> Delay6/1
  "DAFIR v9_0 "/1 -> Delay7/1
  DAFIR v9_0 1/2 -> Logical1/2
  "DAFIR v9_0 "/2 -> Logical1/1
